simulink model "opamps"  (R2018b)
settings: Solver=FixedStepDiscrete  StartTime=0.0  StopTime=10  FixedStep=Ts  RelTol=1e-3
PreLoadFcn:
  | setMatlabPaths
  | Ts = 1e-3
undefined symbols (not defined in the file or in its folder): sigbuilder_block
libraries: Simple_lib x7
settings Model: PauseTimes=1  Creator=billw  LastModifiedBy=billw
settings DataIOCC: SignalLogging=off  DSMLogging=off

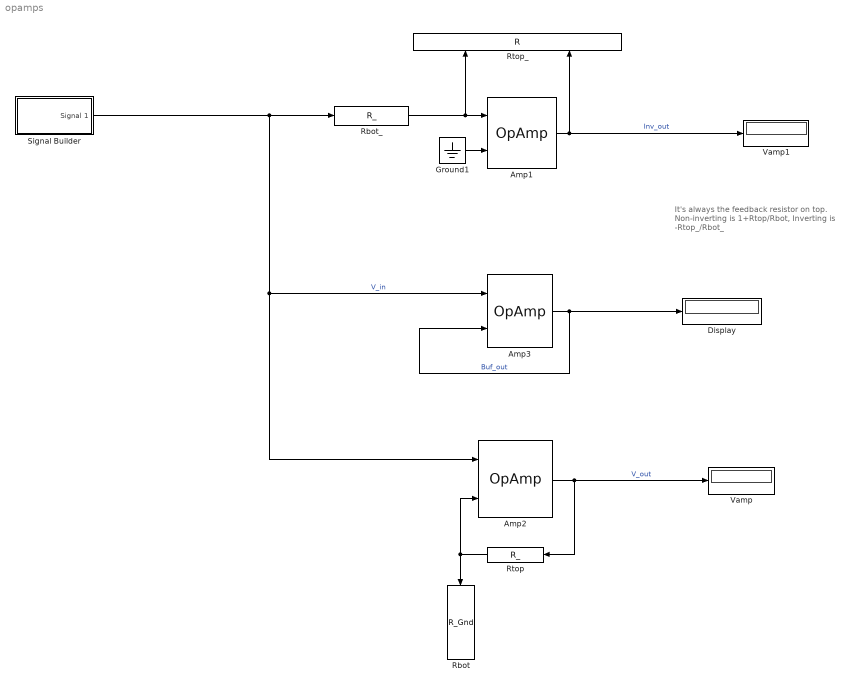
== system opamps ==
  note: It's always the feedback resistor on top.
      | Non-inverting is 1+Rtop/Rbot,
      | Inverting is -Rtop_/Rbot_
  Amp1 : Simple_lib/Electronics/OpAmp  K_op=6
  Amp2 : Simple_lib/Electronics/OpAmp  K_op=6
  Amp3 : Simple_lib/Electronics/OpAmp  K_op=10
  Display : Display
  Ground1 : Ground
  Rbot : Simple_lib/Electronics/R_Gnd  R=1e3
      settings: AttributesFormatString=%<R> Ohm
  Rbot_ : Simple_lib/Electronics/R_  Exponent=3  R=1000
      settings: AttributesFormatString=%<R> Ohm
  Rtop : Simple_lib/Electronics/R_  Exponent=3  R=2700
      settings: AttributesFormatString=%<R> Ohm
  Rtop_ : Simple_lib/Electronics/R  R=4e3
      settings: AttributesFormatString=%<R> Ohms
  Signal Builder : Subsystem  Tag=STV Subsys  LoadFcn=sigbuilder_block('load',[572.4 69.6 550.8 516.6 ]);  StartFcn=sigbuilder_block('start');  StopFcn=sigbuilder_block('stop');  ClipboardFcn=sigbuilder_block('clipboard');  mask(Sigbuilder block){tuvar=[0:10]}
      mask help: Simulink:masks:SigbuilderBlock_MD
      mask init:
      | if ~strcmp(get_param(bdroot(gcbh),'SimulationStatus'),'stopped') tuvar = sigbuilder_block('maskInit'); end
      settings: CopyFcn=sigbuilder_block('copy');  DeleteFcn=sigbuilder_block('delete');  ModelCloseFcn=sigbuilder_block('modelClose');  PreSaveFcn=sigbuilder_block('preSave');  PauseFcn=sigbuilder_block('pause');  ContinueFcn=sigbuilder_block('continue');  NameChangeFcn=sigbuilder_block('namechange');  OpenFcn=sigbuilder_block('open',[572.4 -101.4 550.8 555.6 ]);  CloseFcn=sigbuilder_block('close');
      mask Display: plot(0, 0, 100, 100,[2, 2, 32, 32, 2], [68, 8, 8, 68, 68],[32, 2], [38, 38], [32, 19, 2],[53, 60, 44], [32, 17, 17, 2],[16, 16, 31, 31]);txt = getActiveGroup(gcbh);text(2, 100, txt,'verticalAlignment', 'top');
  Vamp : Display
  Vamp1 : Display
  wires:
  Rtop/1 -> Rbot/1, Amp2/2
  Amp2/1 -> Vamp/1, Rtop/1  "V_out"
  Rbot_/1 -> Rtop_/2, Amp1/2
  Amp1/1 -> Vamp1/1, Rtop_/1  "Inv_out"
  Ground1/1 -> Amp1/1
  Amp3/1 -> Display/1, Amp3/2  "Buf_out"
  Signal Builder/1(Signal 1) -> Amp2/1, Amp3/1, Rbot_/1  "V_in"

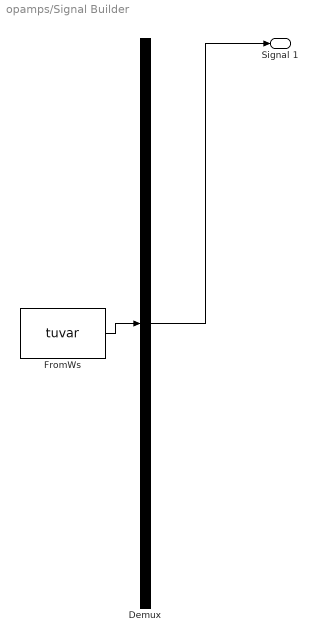
== system opamps/Signal Builder ==
  Demux : Demux  Tag=STV Demux  Outputs=1
  FromWs : FromWorkspace  Tag=STV FromWs  VariableName=tuvar  SampleTime=0
      SigBuilderData=|
      | common.afterFinalStr = 'Extrapolate'
      | common.sampleTime = 0
      | dataSet.timeRange = [0 10]
      | dataSet.name = 'Group 1'
      | sbobj.Groups.Name = 'Group 1'
      | sbobj.Groups.Signals.Name = 'Signal 1'
      | sbobj.Groups.Signals.XData = [0 0.98 2 2 4 4 7.54 10]
      | sbobj.Groups.Signals.YData = [0 2e-07 1 3 3 -2 -1.98 0]
  Signal 1 : Outport  Tag=STV Outport
  wires:
  Demux/1 -> Signal 1/1
  FromWs/1 -> Demux/1
